simulink model "TankSimulink_modell_deg2"  (R2014a)
settings: Solver=ode45  StartTime=0.0  StopTime=800  RelTol=1e-3
values from neighbouring files (symbols this model uses):
  Ar = get(handles.slider_Ar, 'Value')/10000    [TankGui.m]
  cp = get(handles.slider_cp, 'Value')*1000    [TankGui.m]
  g = 9.81    [TankGui.m]
  hoheStart = 0.0001    [TankGui.m]
  Kl = get(handles.slider_Kl, 'Value')    [TankGui.m]
  Kw = get(handles.slider_Kw, 'Value')    [TankGui.m]
  maxFullstand = Vzu^2/Ar^2/(2*g)    [TankGui.m]
  Pel = get(handles.slider_Pel, 'Value')    [TankGui.m]
  rho = get(handles.slider_rho, 'Value')    [TankGui.m]
  thetaSoll = get(handles.slider_Tsoll, 'Value')    [TankGui.m]
  thetaStart = thetaZu    [TankGui.m]
  thetaZu = get(handles.slider_Tzu, 'Value')    [TankGui.m]
  Vzu = get(handles.slider_Vzu, 'Value')/3600    [TankGui.m]
undefined symbols (not defined in the file or in its folder): Alpha, MinHohe, ThetaUm
libraries: simulink x1
settings Model: Creator=Student  LastModifiedBy=Student

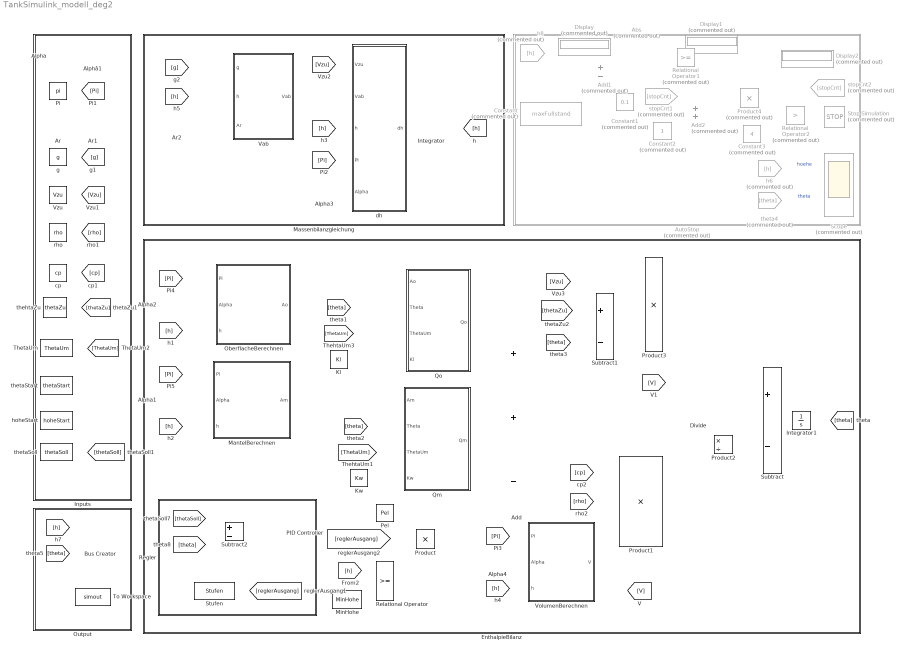
== system TankSimulink_modell_deg2 ==
  Abs : Abs  Commented=on
  Add : Sum  Inputs=++-
  Add1 : Sum  Commented=on  Inputs=+-
  Add2 : Sum  Commented=on
  Alpha : Constant  Value=Alpha
  Ar : Constant  Value=Ar
  AutoStop : Subsystem  Commented=on
  Bus Creator : BusCreator  Inputs=2
  Constant : Constant  Commented=on  Value=maxFullstand
  Constant1 : Constant  Commented=on  Value=0.1
  Constant2 : Constant  Commented=on
  Constant3 : Constant  Commented=on  Value=4
  Display : Display  Commented=on
  Display1 : Display  Commented=on
  Display2 : Display  Commented=on
  Divide : Product  Inputs=*/
  EnthalpieBilanz : Subsystem
  Inputs : Subsystem
  Integrator : Integrator  InitialCondition=hoheStart
  Integrator1 : Integrator  InitialCondition=thetaStart
  Kl : Constant  Value=Kl
  Kw : Constant  Value=Kw
  MantelBerechnen : Subsystem
  Massenbilanzgleichung : Subsystem
  MinHohe : Constant  Value=MinHohe
  OberflacheBerechnen : Subsystem
  Output : Subsystem
  PID Controller : simulink/Continuous/PID Controller  Controller=PI  TimeDomain=Continuous-time  SampleTime=1  IntegratorMethod=Forward Euler  FilterMethod=Forward Euler  Form=Parallel  P=1.5  I=0.1  D=0  N=100  InitialConditionSource=internal  InitialConditionForIntegrator=0  InitialConditionForFilter=0  ExternalReset=none  LimitOutput=on  UpperSaturationLimit=1  LowerSaturationLimit=0  LinearizeAsGain=off  AntiWindupMode=back-calculation  Kb=1  TrackingMode=off  Kt=1  PParamMin=[]  PParamMax=[]  IParamMin=[]  IParamMax=[]  DParamMin=[]  DParamMax=[]  NParamMin=[]  NParamMax=[]  KbParamMin=[]  KbParamMax=[]  KtParamMin=[]  KtParamMax=[]  POutMin=[]  POutMax=[]  IOutMin=[]  IOutMax=[]  DOutMin=[]  DOutMax=[]  NOutMin=[]  NOutMax=[]  KbOutMin=[]  KbOutMax=[]  KtOutMin=[]  KtOutMax=[]  IntegratorOutMin=[]  IntegratorOutMax=[]  FilterOutMin=[]  FilterOutMax=[]  SumOutMin=[]  SumOutMax=[]  SumI1OutMin=[]  SumI1OutMax=[]  SumI2OutMin=[]  SumI2OutMax=[]  SumI3OutMin=[]  SumI3OutMax=[]  SumDOutMin=[]  SumDOutMax=[]  SaturationOutMin=[]  SaturationOutMax=[]  IntegratorContinuousStateAttributes=''  IntegratorStateMustResolveToSignalObject=off  IntegratorRTWStateStorageClass=Auto  FilterContinuousStateAttributes=''  FilterStateMustResolveToSignalObject=off  FilterRTWStateStorageClass=Auto
  Pel : Constant  Value=Pel
  Pi : Constant  Value=pi
  Product : Product  Inputs=3
  Product1 : Product  Inputs=3
  Product2 : Product  Inputs=*/
  Product3 : Product
  Product4 : Product  Commented=on
  Qm : Subsystem
  Qo : Subsystem
  Regler : Subsystem
  Relational Operator : RelationalOperator  OutDataTypeStr=boolean
  Relational Operator1 : RelationalOperator  Commented=on  OutDataTypeStr=boolean
  Relational Operator2 : RelationalOperator  Commented=on  Operator=>  OutDataTypeStr=boolean
  Scope : Scope  Commented=on  NumInputPorts=2
      settings: ShowLegends=on  YMin=2.77556e-17~20  YMax=1.1~50
  Stop Simulation : Stop  Commented=on
  Stufen : MATLABFcn  MATLABFcn=Stufen
  Subtract : Sum  Inputs=+-
  Subtract1 : Sum  Inputs=+-
  Subtract2 : Sum  Inputs=+-
  ThetaUm : Constant  Value=ThetaUm
  To Workspace : ToWorkspace  VariableName=simout  SaveFormat=Structure With Time  SampleTime=-1
  Vab : Subsystem
  VolumenBerechnen : Subsystem
  Vzu : Constant  Value=Vzu
  cp : Constant  Value=cp
  "dh " : Subsystem
  g : Constant  Value=g
  h6 : From  Commented=on  GotoTag=h
  h8 : From  Commented=on  GotoTag=h
  hoheStart : Constant  Value=hoheStart
  rho : Constant  Value=rho
  stopCnt1 : From  Commented=on  GotoTag=stopCnt
  stopCnt2 : Goto  Commented=on  GotoTag=stopCnt
  thehtaZu : Constant  Value=thetaZu
  theta4 : From  Commented=on  GotoTag=theta
  thetaSoll : Constant  Value=thetaSoll
  thetaStart : Constant  Value=thetaStart
  wires:
  OberflacheBerechnen/1(Ao) -> Qo/1(Ao)
  MantelBerechnen/1(Am) -> Qm/1(Am)
  Kw/1 -> Qm/4(Kw)
  Kl/1 -> Qo/4(Kl)
  Vab/1(Vab) -> "dh "/2(Vab)
  Alpha/1 -> [Alpha]
  Pi/1 -> [Pi]
  Ar/1 -> [Ar]
  [h] -> Vab/2(h)
  [h] -> "dh "/3(h)
  "dh "/1(dh) -> Integrator/1
  Integrator/1 -> [h]
  [Pi] -> "dh "/4(Pi)
  [Ar] -> Vab/3(Ar)
  [g] -> Vab/1(g)
  g/1 -> [g]
  Vzu/1 -> [Vzu]
  [Vzu] -> "dh "/1(Vzu)
  [Alpha] -> "dh "/5(Alpha)
  Qo/1(Qo) -> Add/1
  Qm/1(Qm) -> Add/2
  [h] -> Relational Operator/1
  MinHohe/1 -> Relational Operator/2
  Product/1 -> Add/3
  VolumenBerechnen/1(V) -> [V], Product1/3
  rho/1 -> [rho]
  [rho] -> Product1/2
  cp/1 -> [cp]
  [cp] -> Product1/1
  Add/1 -> Product2/1
  Product1/1 -> Product2/2
  [Pi] -> VolumenBerechnen/1(Pi)
  [Alpha] -> VolumenBerechnen/2(Alpha)
  [h] -> VolumenBerechnen/3(h)
  [Pi] -> OberflacheBerechnen/1(Pi)
  [Pi] -> MantelBerechnen/1(Pi)
  [Alpha] -> MantelBerechnen/2(Alpha)
  [Alpha] -> OberflacheBerechnen/2(Alpha)
  [h] -> OberflacheBerechnen/3(h)
  [h] -> MantelBerechnen/3(h)
  ThetaUm/1 -> [ThetaUm]
  [ThetaUm] -> Qo/3(ThetaUm)
  [ThetaUm] -> Qm/3(ThetaUm)
  Product2/1 -> Subtract/2
  Subtract/1 -> Integrator1/1
  Integrator1/1 -> [theta]
  [theta] -> Qo/2(Theta)
  [theta] -> Qm/2(Theta)
  [theta] -> Subtract1/2
  thehtaZu/1 -> [thetaZu]
  [thetaZu] -> Subtract1/1
  Subtract1/1 -> Product3/2
  [Vzu] -> Product3/1
  Product3/1 -> Divide/1
  [V] -> Divide/2
  Divide/1 -> Subtract/1
  theta4/1 -> Scope/2  "theta"
  h6/1 -> Scope/1  "hoehe"
  thetaSoll/1 -> [thetaSoll]
  Pel/1 -> Product/1
  Subtract2/1 -> PID Controller/1
  [thetaSoll] -> Subtract2/1
  [theta] -> Subtract2/2
  Relational Operator/1 -> Product/3
  Bus Creator/1 -> To Workspace/1
  [h] -> Bus Creator/1
  [theta] -> Bus Creator/2
  PID Controller/1 -> Stufen/1
  Stufen/1 -> [reglerAusgang]
  [reglerAusgang] -> Product/2
  Relational Operator1/1 -> Product4/1
  Constant2/1 -> Add2/2
  stopCnt1/1 -> Add2/1
  Add2/1 -> Product4/2
  Product4/1 -> Relational Operator2/1, Display2/1, stopCnt2/1
  Constant3/1 -> Relational Operator2/2
  Relational Operator2/1 -> Stop Simulation/1
  Constant/1 -> Add1/2
  Constant1/1 -> Relational Operator1/2
  Add1/1 -> Abs/1
  Abs/1 -> Display1/1, Relational Operator1/1
  h8/1 -> Display/1, Add1/1

== system TankSimulink_modell_deg2/AutoStop ==

== system TankSimulink_modell_deg2/EnthalpieBilanz ==

== system TankSimulink_modell_deg2/Inputs ==

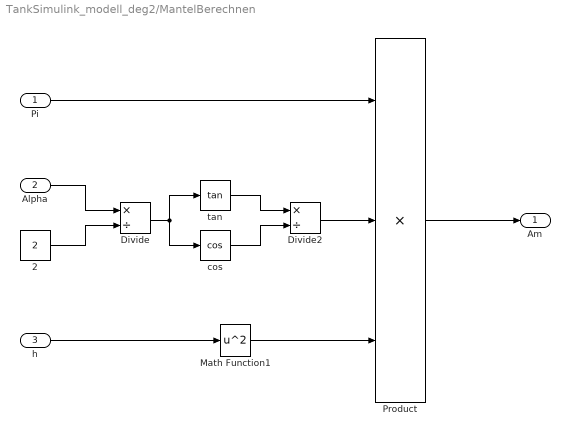
== system TankSimulink_modell_deg2/MantelBerechnen ==
  Pi : Inport
  Alpha : Inport  Port=2
  h : Inport  Port=3
  2 : Constant  Value=2
  Divide : Product  Inputs=*/
  Divide2 : Product  Inputs=*/
  Math Function1 : Math  Operator=square  SaturateOnIntegerOverflow=on
  Product : Product  Inputs=3
  cos : Trigonometry  Operator=cos
  tan : Trigonometry  Operator=tan
  Am : Outport
  wires:
  Pi/1 -> Product/1
  Alpha/1 -> Divide/1
  2/1 -> Divide/2
  Divide/1 -> cos/1, tan/1
  Math Function1/1 -> Product/3
  h/1 -> Math Function1/1
  tan/1 -> Divide2/1
  cos/1 -> Divide2/2
  Divide2/1 -> Product/2
  Product/1 -> Am/1

== system TankSimulink_modell_deg2/Massenbilanzgleichung ==

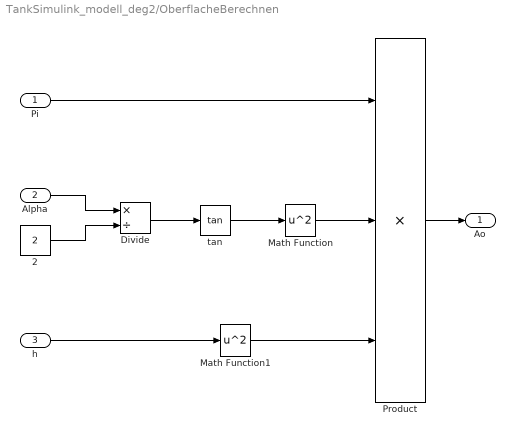
== system TankSimulink_modell_deg2/OberflacheBerechnen ==
  Pi : Inport
  Alpha : Inport  Port=2
  h : Inport  Port=3
  2 : Constant  Value=2
  Divide : Product  Inputs=*/
  Math Function : Math  Operator=square  SaturateOnIntegerOverflow=on
  Math Function1 : Math  Operator=square  SaturateOnIntegerOverflow=on
  Product : Product  Inputs=3
  tan : Trigonometry  Operator=tan
  Ao : Outport
  wires:
  Pi/1 -> Product/1
  Alpha/1 -> Divide/1
  2/1 -> Divide/2
  Math Function/1 -> Product/2
  Divide/1 -> tan/1
  tan/1 -> Math Function/1
  Math Function1/1 -> Product/3
  h/1 -> Math Function1/1
  Product/1 -> Ao/1

== system TankSimulink_modell_deg2/Output ==

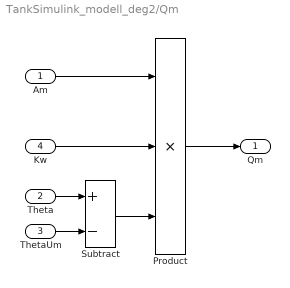
== system TankSimulink_modell_deg2/Qm ==
  Am : Inport
  Theta : Inport  Port=2
  ThetaUm : Inport  Port=3
  Kw : Inport  Port=4
  Product : Product  Inputs=3
  Subtract : Sum  Inputs=+-
  Qm : Outport
  wires:
  Theta/1 -> Subtract/1
  ThetaUm/1 -> Subtract/2
  Subtract/1 -> Product/3
  Kw/1 -> Product/2
  Am/1 -> Product/1
  Product/1 -> Qm/1

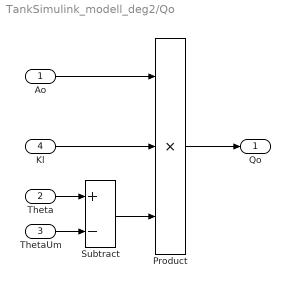
== system TankSimulink_modell_deg2/Qo ==
  Ao : Inport
  Theta : Inport  Port=2
  ThetaUm : Inport  Port=3
  Kl : Inport  Port=4
  Product : Product  Inputs=3
  Subtract : Sum  Inputs=+-
  Qo : Outport
  wires:
  Theta/1 -> Subtract/1
  ThetaUm/1 -> Subtract/2
  Subtract/1 -> Product/3
  Kl/1 -> Product/2
  Ao/1 -> Product/1
  Product/1 -> Qo/1

== system TankSimulink_modell_deg2/Regler ==

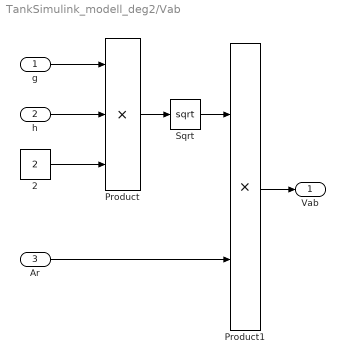
== system TankSimulink_modell_deg2/Vab ==
  g : Inport
  h : Inport  Port=2
  Ar : Inport  Port=3
  2 : Constant  Value=2
  Product : Product  Inputs=3
  Product1 : Product
  Sqrt : Sqrt  SaturateOnIntegerOverflow=on
  Vab : Outport
  wires:
  g/1 -> Product/1
  h/1 -> Product/2
  2/1 -> Product/3
  Product/1 -> Sqrt/1
  Sqrt/1 -> Product1/1
  Ar/1 -> Product1/2
  Product1/1 -> Vab/1

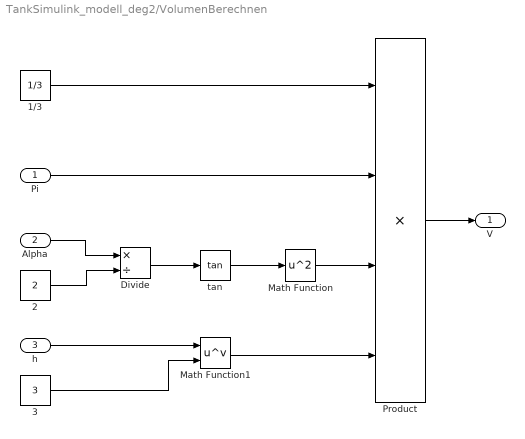
== system TankSimulink_modell_deg2/VolumenBerechnen ==
  Pi : Inport
  Alpha : Inport  Port=2
  h : Inport  Port=3
  1/3 : Constant  Value=1/3
  2 : Constant  Value=2
  3 : Constant  Value=3
  Divide : Product  Inputs=*/
  Math Function : Math  Operator=square  SaturateOnIntegerOverflow=on
  Math Function1 : Math  Operator=pow  SaturateOnIntegerOverflow=on
  Product : Product  Inputs=4
  tan : Trigonometry  Operator=tan
  V : Outport
  wires:
  Alpha/1 -> Divide/1
  2/1 -> Divide/2
  Math Function/1 -> Product/3
  Divide/1 -> tan/1
  tan/1 -> Math Function/1
  Math Function1/1 -> Product/4
  h/1 -> Math Function1/1
  Product/1 -> V/1
  1/3/1 -> Product/1
  Pi/1 -> Product/2
  3/1 -> Math Function1/2

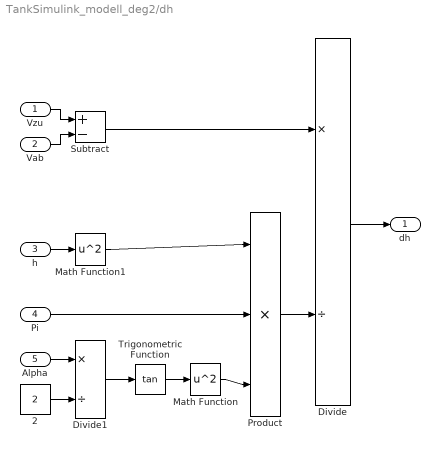
== system TankSimulink_modell_deg2/dh  ==
  Vzu : Inport
  Vab : Inport  Port=2
  h : Inport  Port=3
  Pi : Inport  Port=4
  Alpha : Inport  Port=5
  2 : Constant  Value=2
  Divide : Product  Inputs=*/
  Divide1 : Product  Inputs=*/
  Math Function : Math  Operator=square  SaturateOnIntegerOverflow=on
  Math Function1 : Math  Operator=square  SaturateOnIntegerOverflow=on
  Product : Product  Inputs=3
  Subtract : Sum  Inputs=+-
  Trigonometric Function : Trigonometry  Operator=tan  ApproximationMethod=CORDIC
  dh : Outport
  wires:
  Vzu/1 -> Subtract/1
  Vab/1 -> Subtract/2
  Alpha/1 -> Divide1/1
  2/1 -> Divide1/2
  Divide1/1 -> Trigonometric Function/1
  Trigonometric Function/1 -> Math Function/1
  h/1 -> Math Function1/1
  Math Function/1 -> Product/3
  Pi/1 -> Product/2
  Math Function1/1 -> Product/1
  Product/1 -> Divide/2
  Subtract/1 -> Divide/1
  Divide/1 -> dh/1
